simulink model "benchmark_model"  (R2021a)
settings: Solver=ode1  StartTime=0.0  StopTime=Tend  FixedStep=0.0001  MaxStep=0.1  MinStep=0.0001  AbsTol=0.01  EnableMultiTasking=on
undefined symbols (not defined in the file): A1, A2, AL, AM0, AREA, BORE, C_EGR, c_f, c_T, CAIR, cCO, cCO2, cH2, cH2O, cHC, cN2, CO, CO2, cO2, DEN0, DiscIntNeverNeededParam, EGR_dia, EGR_sk, EX_AREA, EX_M_AR, EXO, FD0, FOM, FR0, FR_C1, FR_C2, FR_C3, FR_C4, FR_C5, H2, H2O, HC, INC, INO, KET, Kex, Kh, MAS0, MCh, MHC, MN2, MO2, MOLcylT, N2, O2, PR0, R150, Rabs, SPEC, TBORE, Th_HC, Th_knock, THEX, THIN, TM0 ... (+9)
libraries: pid_lib x1
(part 4 of 6)

== system benchmark_model/ENGINE/engine_s/cylinders/cyl1/cyl/heat_trans/cyl_wall ==
  qw_v : Inport
  Tw0 : Inport  Port=2
  Gain1 : Gain  Gain=1/2.5
  Gain2 : Gain  Gain=1.0
  Gain5 : Gain  Gain=3.0
  Integrator : Integrator  InitialConditionSource=external
  Subtract : Sum  Inputs=-+
  Subtract2 : Sum  Inputs=+-
  Tw : Outport
  wires:
  Tw0/1 -> Subtract2/2, Integrator/2
  Subtract/1 -> Gain1/1
  Gain1/1 -> Integrator/1
  Integrator/1 -> Tw/1, Subtract2/1
  Gain2/1 -> Subtract/2
  Subtract2/1 -> Gain5/1
  Gain5/1 -> Subtract/1
  qw_v/1 -> Gain2/1

== system benchmark_model/ENGINE/engine_s/cylinders/cyl1/cyl/knock_Integral/Subsystem1 ==
  pc : Inport
  rps : Inport  Port=2
  Tc : Inport  Port=3
  rad : Inport  Port=4
  Constant1 : Constant  Value=0
  Constant2 : Constant  Value=FR_C1
  Constant3 : Constant
  Constant4 : Constant  Value=(540+INC)*pi/180
  Constant5 : Constant  Value=(180-EXO)*pi/180
  Divide1 : Product  Inputs=3
  Divide2 : Product  Inputs=*/
  Fcn : Fcn  Expr=-FR_C2*(-FR_C4*u+FR_C5)
  Gain : Gain  Gain=0.001
  Integrator : Integrator  ExternalReset=rising
  Math Function : Math  Operator=pow  SignedPower=on  SaturateOnIntegerOverflow=on
  Memory : Memory
  Relational Operator1 : RelationalOperator  Operator=<=  OutDataTypeStr=boolean  RndMeth=Nearest
  Relational Operator2 : RelationalOperator  OutDataTypeStr=boolean  RndMeth=Nearest
  Saturation : Saturate  UpperLimit=inf  LowerLimit=1.0e-16
  Subsystem : Subsystem
  Switch : Switch  Threshold=0.5
  cal_unburned_temp : Subsystem
  ki : Outport
  wires:
  pc/1 -> Saturation/1
  Fcn/1 -> Math Function/2
  Math Function/1 -> Divide1/2
  Constant2/1 -> Divide1/1
  Subsystem/1(Out1) -> Divide1/3
  Divide1/1 -> Divide2/2
  Constant3/1 -> Divide2/1
  Divide2/1 -> Integrator/1
  Tc/1 -> cal_unburned_temp/2(Tc)
  Memory/1 -> Integrator/2
  cal_unburned_temp/1(Tu) -> Subsystem/1(Tu)
  Gain/1 -> Math Function/1
  Integrator/1 -> Switch/1
  Switch/1 -> ki/1
  Constant1/1 -> Switch/3
  rad/1 -> Relational Operator1/1, Relational Operator2/1
  Constant4/1 -> Relational Operator2/2
  Relational Operator2/1 -> cal_unburned_temp/3(trg_inc), Memory/1
  Constant5/1 -> Relational Operator1/2
  Relational Operator1/1 -> Switch/2
  rps/1 -> Fcn/1
  Saturation/1 -> cal_unburned_temp/1(Pc), Gain/1

== system benchmark_model/ENGINE/engine_s/cylinders/cyl1/cyl/knock_Integral/Triggered Subsystem ==
  QA_max : Inport
  QA : Inport  Port=2
  Trigger : TriggerPort  VariantControl=(inherit)
  Constant1 : Constant  Value=0
  Constant2 : Constant  Value=1.0e-9
  Relational Operator : RelationalOperator  OutDataTypeStr=boolean  RndMeth=Nearest
  Subtract : Sum  Inputs=+-
  Switch : Switch  Threshold=0.5
  AI_Q : Outport  InitialOutput=0
  wires:
  QA/1 -> Subtract/2
  QA_max/1 -> Subtract/1
  Constant1/1 -> Switch/3
  Switch/1 -> AI_Q/1
  Subtract/1 -> Relational Operator/1, Switch/1
  Relational Operator/1 -> Switch/2
  Constant2/1 -> Relational Operator/2

== system benchmark_model/ENGINE/engine_s/cylinders/cyl1/cyl/ramining ratio of fuel/Triggered Subsystem ==
  QA : Inport
  Trigger : TriggerPort  VariantControl=(inherit)
  Constant : Constant
  Constant1 : Constant  Value=0
  Constant2 : Constant  Value=1.0e-9
  Relational Operator : RelationalOperator  OutDataTypeStr=boolean  RndMeth=Nearest
  Subtract : Sum  Inputs=+-
  Switch : Switch  Threshold=0.5
  AI_Q : Outport  InitialOutput=0
  wires:
  Constant2/1 -> Relational Operator/2
  Relational Operator/1 -> Switch/2
  Subtract/1 -> Switch/1, Relational Operator/1
  Switch/1 -> AI_Q/1
  Constant1/1 -> Switch/3
  Constant/1 -> Subtract/1
  QA/1 -> Subtract/2

== system benchmark_model/ENGINE/engine_s/cylinders/cyl1/cyl/unburnt_gass/add_fuel1 ==
  Nfuel : Inport
  mol : Inport  Port=2
  Add : Sum
  Demux : Demux  Outputs=7
  Mux : Mux  Inputs=7
  add_fuel : Outport
  wires:
  Demux/2 -> Mux/2
  Demux/3 -> Mux/3
  Demux/4 -> Mux/4
  Demux/5 -> Mux/5
  Demux/6 -> Mux/6
  Demux/7 -> Mux/7
  mol/1 -> Demux/1
  Mux/1 -> add_fuel/1
  Demux/1 -> Add/2
  Add/1 -> Mux/1
  Nfuel/1 -> Add/1

== system benchmark_model/ENGINE/engine_s/cylinders/cyl1/cyl/unburnt_gass/init&trig ==
  trig : Inport
  value : Inport  Port=2
  Demux : Demux  Outputs=7
  Mux : Mux  Inputs=7
  qChart : Stateflow chart  TreatAsAtomicUnit=on
  init : Outport
  wires:
  value/1 -> Demux/1
  Demux/1 -> qChart/1(sl_in1)
  Demux/2 -> qChart/2(sl_in2)
  Demux/3 -> qChart/3(sl_in3)
  Demux/4 -> qChart/4(sl_in4)
  Demux/5 -> qChart/5(sl_in5)
  Demux/6 -> qChart/6(sl_in6)
  Demux/7 -> qChart/7(sl_in7)
  qChart/7(sl_out7) -> Mux/7
  qChart/1(sl_out1) -> Mux/1
  qChart/2(sl_out2) -> Mux/2
  qChart/3(sl_out3) -> Mux/3
  qChart/4(sl_out4) -> Mux/4
  qChart/5(sl_out5) -> Mux/5
  qChart/6(sl_out6) -> Mux/6
  Mux/1 -> init/1
  trig/1 -> qChart/Trigger

== system benchmark_model/ENGINE/engine_s/cylinders/cyl1/selectors/selector/mod720(u,4*pi) ==
  u : Inport
  Constant7 : Constant  Value=4*pi
  Math Function : Math  Operator=mod  SignedPower=on  SaturateOnIntegerOverflow=on
  y : Outport
  wires:
  Math Function/1 -> y/1
  u/1 -> Math Function/1
  Constant7/1 -> Math Function/2

== system benchmark_model/ENGINE/engine_s/cylinders/cyl2/cyl/Energy_Int/dvol ==
  rad : Inport
  rps : Inport  Port=2
  Product : Product  RndMeth=Zero
  func_d_cylvol(u,SPEC) : Subsystem
  dvol : Outport
  wires:
  func_d_cylvol(u,SPEC)/1(Out1) -> Product/1
  rad/1 -> func_d_cylvol(u,SPEC)/1(In1)
  Product/1 -> dvol/1
  rps/1 -> Product/2

== system benchmark_model/ENGINE/engine_s/cylinders/cyl2/cyl/cal_cyl_state/cal_state ==
  note: p/d = R T
      | T = P/d/R
  m : Inport
  n : Inport  Port=2
  f : Inport  Port=3
  E : Inport  Port=4
  vol : Inport  Port=5
  Fcn : Fcn  Expr=2/u[1]*u[3]/u[2]
  Fcn1 : Fcn  Expr=u[3]/u[1]/(Rabs/u[2])
  Mux : Mux  Inputs=3
  Mux1 : Mux
  Mux2 : Mux  Inputs=3
  Product1 : Product  Inputs=/*  RndMeth=Zero
  Product2 : Product  Inputs=*/  RndMeth=Zero
  Product3 : Product  Inputs=*/  RndMeth=Zero
  pc : Outport  InitialOutput=0
  tc : Outport  Port=2  InitialOutput=0
  cyl_st : Outport  Port=3  InitialOutput=0
  wires:
  Fcn1/1 -> tc/1
  E/1 -> Mux/3
  f/1 -> Product1/2
  n/1 -> Product2/2, Product1/1
  m/1 -> Product3/1, Product2/1
  Mux2/1 -> Fcn1/1
  Product3/1 -> Mux1/1, Mux2/1  "dens"
  Product2/1 -> Mux1/3, Mux2/2  "gas_c"
  Product1/1 -> Mux1/4, Mux/1  "deg of freedom"
  vol/1 -> Product3/2, Mux/2
  Mux1/1 -> cyl_st/1
  Mux/1 -> Fcn/1
  Fcn/1 -> pc/1, Mux2/3, Mux1/2  "pres"

== system benchmark_model/ENGINE/engine_s/cylinders/cyl2/cyl/crank/Subsystem1 ==
  trig_inj : Inport
  fc : Inport  Port=2
  N/s : Inport  Port=3
  Gain : Gain  Gain=MHC
  Integrator : Integrator  ExternalReset=rising
  Product : Product
  Relational Operator1 : RelationalOperator  OutDataTypeStr=boolean  RndMeth=Nearest
  N_fuel : Outport
  wires:
  Gain/1 -> Integrator/1
  N/s/1 -> Gain/1, Product/2
  fc/1 -> Relational Operator1/1
  Relational Operator1/1 -> Product/1
  Integrator/1 -> Relational Operator1/2
  Product/1 -> N_fuel/1
  trig_inj/1 -> Integrator/2

== system benchmark_model/ENGINE/engine_s/cylinders/cyl2/cyl/crank/inj_start ==
  rad : Inport
  Constant3 : Constant  Value=(360-INO+1)*pi/180
  Relational Operator2 : RelationalOperator  OutDataTypeStr=boolean  RndMeth=Nearest
  trig_inj : Outport
  wires:
  Relational Operator2/1 -> trig_inj/1
  rad/1 -> Relational Operator2/1
  Constant3/1 -> Relational Operator2/2

== system benchmark_model/ENGINE/engine_s/cylinders/cyl2/cyl/crank/mol_flow_rate ==
  rps : Inport
  Constant1 : Constant  Value=0.50*pi
  Constant2 : Constant  Value=MHC
  Divide2 : Product  Inputs=*/
  Divide3 : Product  Inputs=*/
  Divide4 : Product  Inputs=*/
  inje/s : Constant  Value=(DEN0*VH/14.5)
  N/s : Outport
  wires:
  Divide2/1 -> Divide3/1
  Divide4/1 -> Divide2/2
  rps/1 -> Divide4/2
  Constant1/1 -> Divide4/1
  inje/s/1 -> Divide2/1
  Divide3/1 -> N/s/1
  Constant2/1 -> Divide3/2

== system benchmark_model/ENGINE/engine_s/cylinders/cyl2/cyl/frame/Init_cyl_gas ==
  tr_inc : Inport
  mol_s : Inport  Port=2
  capture_cyl_state : Subsystem  TreatAsAtomicUnit=on
  init_gas : Outport
  Qmax : Outport  Port=2
  b_comp : Outport  Port=3
  af : Outport  Port=4
  wires:
  tr_inc/1 -> capture_cyl_state/Trigger
  capture_cyl_state/4(af) -> af/1
  capture_cyl_state/1(Qmax) -> Qmax/1
  mol_s/1 -> capture_cyl_state/1(cyl_gas)
  capture_cyl_state/2(b_comp) -> b_comp/1
  capture_cyl_state/3(init_gas) -> init_gas/1

== system benchmark_model/ENGINE/engine_s/cylinders/cyl2/cyl/frame/ratio_burnt1 ==
  rps : Inport
  rad : Inport  Port=2
  AF : Inport  Port=3
  KL : Inport  Port=4
  SA : Inport  Port=5
  EGR : Inport  Port=6
  VT : Inport  Port=7
  Add : Sum
  Constant : Constant  Value=(180-EXO-1)*pi/180+pi
  Constant1 : Constant  Value=0
  Constant2 : Constant  Value=pi
  Constant3 : Constant  Value=0
  Product : Product  RndMeth=Zero
  Relational Operator : RelationalOperator  Operator=<  OutDataTypeStr=boolean  RndMeth=Nearest
  Switch : Switch  Threshold=0.5
  Switch1 : Switch  Threshold=0.5
  mod720(u,4*pi) : Subsystem
  murnt_ratio : Subsystem
  burnt_ratio : Outport  PortDimensions=1  InitialOutput=0
  QR : Outport  Port=2  PortDimensions=1  InitialOutput=0
  Q : Outport  Port=3  PortDimensions=1  InitialOutput=0
  wires:
  VT/1 -> murnt_ratio/7(VT)
  Switch1/1 -> Q/1
  Constant3/1 -> Switch1/3
  murnt_ratio/2(Q) -> Switch1/1
  Constant2/1 -> Add/1
  rad/1 -> Add/2
  Add/1 -> mod720(u,4*pi)/1(u)
  EGR/1 -> murnt_ratio/6(EGR)
  Product/1 -> burnt_ratio/1
  Switch/1 -> QR/1, Product/1
  Constant1/1 -> Switch/3
  Relational Operator/1 -> Switch/2, Switch1/2
  Constant/1 -> Relational Operator/2
  SA/1 -> murnt_ratio/2(SA)
  KL/1 -> murnt_ratio/4(KL)
  AF/1 -> murnt_ratio/5(AF)
  rps/1 -> Product/2, murnt_ratio/3(rps)
  mod720(u,4*pi)/1(y) -> Relational Operator/1, murnt_ratio/1(u)
  murnt_ratio/1(q) -> Switch/1

== system benchmark_model/ENGINE/engine_s/cylinders/cyl2/cyl/heat_trans/cal_cyl_ar ==
  vol : Inport
  Add2 : Sum
  Constant1 : Constant  Value=2*pi*BORE
  Constant2 : Constant  Value=AREA
  Gain1 : Gain  Gain=2
  Product1 : Product  Inputs=*/  RndMeth=Zero
  Product2 : Product  RndMeth=Zero
  cyl_ar : Outport
  wires:
  Product2/1 -> Add2/1
  Constant1/1 -> Product2/1
  Product1/1 -> Product2/2
  Add2/1 -> cyl_ar/1
  vol/1 -> Product1/1
  Gain1/1 -> Add2/2
  Constant2/1 -> Gain1/1, Product1/2

== system benchmark_model/ENGINE/engine_s/cylinders/cyl2/cyl/heat_trans/cal_qw ==
  pc : Inport
  rps : Inport  Port=2
  Tg : Inport  Port=3
  Tw : Inport  Port=4
  Fcn : Fcn  Expr=(u(1)*u(2))^0.786*u(3)^(-0.525)*(u(3)-u(4))
  Mux3 : Mux
  Saturation : Saturate  UpperLimit=inf  LowerLimit=1.0e-16
  qw : Outport
  wires:
  Saturation/1 -> Fcn/1
  Tg/1 -> Mux3/3
  rps/1 -> Mux3/2
  pc/1 -> Mux3/1
  Tw/1 -> Mux3/4
  Fcn/1 -> qw/1
  Mux3/1 -> Saturation/1

== system benchmark_model/ENGINE/engine_s/cylinders/cyl2/cyl/heat_trans/cyl_wall ==
  qw_v : Inport
  Tw0 : Inport  Port=2
  Gain1 : Gain  Gain=1/2.5
  Gain2 : Gain  Gain=1.0
  Gain5 : Gain  Gain=3.0
  Integrator : Integrator  InitialConditionSource=external
  Subtract : Sum  Inputs=-+
  Subtract2 : Sum  Inputs=+-
  Tw : Outport
  wires:
  qw_v/1 -> Gain2/1
  Gain5/1 -> Subtract/1
  Subtract2/1 -> Gain5/1
  Gain2/1 -> Subtract/2
  Integrator/1 -> Subtract2/1, Tw/1
  Gain1/1 -> Integrator/1
  Subtract/1 -> Gain1/1
  Tw0/1 -> Integrator/2, Subtract2/2

== system benchmark_model/ENGINE/engine_s/cylinders/cyl2/cyl/knock_Integral/Subsystem1 ==
  pc : Inport
  rps : Inport  Port=2
  Tc : Inport  Port=3
  rad : Inport  Port=4
  Constant1 : Constant  Value=0
  Constant2 : Constant  Value=FR_C1
  Constant3 : Constant
  Constant4 : Constant  Value=(540+INC)*pi/180
  Constant5 : Constant  Value=(180-EXO)*pi/180
  Divide1 : Product  Inputs=3
  Divide2 : Product  Inputs=*/
  Fcn : Fcn  Expr=-FR_C2*(-FR_C4*u+FR_C5)
  Gain : Gain  Gain=0.001
  Integrator : Integrator  ExternalReset=rising
  Math Function : Math  Operator=pow  SignedPower=on  SaturateOnIntegerOverflow=on
  Memory : Memory
  Relational Operator1 : RelationalOperator  Operator=<=  OutDataTypeStr=boolean  RndMeth=Nearest
  Relational Operator2 : RelationalOperator  OutDataTypeStr=boolean  RndMeth=Nearest
  Saturation : Saturate  UpperLimit=inf  LowerLimit=1.0e-16
  Subsystem : Subsystem
  Switch : Switch  Threshold=0.5
  cal_unburned_temp : Subsystem
  ki : Outport
  wires:
  Saturation/1 -> Gain/1, cal_unburned_temp/1(Pc)
  rps/1 -> Fcn/1
  Relational Operator1/1 -> Switch/2
  Constant5/1 -> Relational Operator1/2
  Relational Operator2/1 -> Memory/1, cal_unburned_temp/3(trg_inc)
  Constant4/1 -> Relational Operator2/2
  rad/1 -> Relational Operator2/1, Relational Operator1/1
  Constant1/1 -> Switch/3
  Switch/1 -> ki/1
  Integrator/1 -> Switch/1
  Gain/1 -> Math Function/1
  cal_unburned_temp/1(Tu) -> Subsystem/1(Tu)
  Memory/1 -> Integrator/2
  Tc/1 -> cal_unburned_temp/2(Tc)
  Divide2/1 -> Integrator/1
  Constant3/1 -> Divide2/1
  Divide1/1 -> Divide2/2
  Subsystem/1(Out1) -> Divide1/3
  Constant2/1 -> Divide1/1
  Math Function/1 -> Divide1/2
  Fcn/1 -> Math Function/2
  pc/1 -> Saturation/1

== system benchmark_model/ENGINE/engine_s/cylinders/cyl2/cyl/knock_Integral/Triggered Subsystem ==
  QA_max : Inport
  QA : Inport  Port=2
  Trigger : TriggerPort  VariantControl=(inherit)
  Constant1 : Constant  Value=0
  Constant2 : Constant  Value=1.0e-9
  Relational Operator : RelationalOperator  OutDataTypeStr=boolean  RndMeth=Nearest
  Subtract : Sum  Inputs=+-
  Switch : Switch  Threshold=0.5
  AI_Q : Outport  InitialOutput=0
  wires:
  Constant2/1 -> Relational Operator/2
  Relational Operator/1 -> Switch/2
  Subtract/1 -> Switch/1, Relational Operator/1
  Switch/1 -> AI_Q/1
  Constant1/1 -> Switch/3
  QA_max/1 -> Subtract/1
  QA/1 -> Subtract/2

== system benchmark_model/ENGINE/engine_s/cylinders/cyl2/cyl/ramining ratio of fuel/Triggered Subsystem ==
  QA : Inport
  Trigger : TriggerPort  VariantControl=(inherit)
  Constant : Constant
  Constant1 : Constant  Value=0
  Constant2 : Constant  Value=1.0e-9
  Relational Operator : RelationalOperator  OutDataTypeStr=boolean  RndMeth=Nearest
  Subtract : Sum  Inputs=+-
  Switch : Switch  Threshold=0.5
  AI_Q : Outport  InitialOutput=0
  wires:
  QA/1 -> Subtract/2
  Constant/1 -> Subtract/1
  Constant1/1 -> Switch/3
  Switch/1 -> AI_Q/1
  Subtract/1 -> Relational Operator/1, Switch/1
  Relational Operator/1 -> Switch/2
  Constant2/1 -> Relational Operator/2

== system benchmark_model/ENGINE/engine_s/cylinders/cyl2/cyl/unburnt_gass/add_fuel1 ==
  Nfuel : Inport
  mol : Inport  Port=2
  Add : Sum
  Demux : Demux  Outputs=7
  Mux : Mux  Inputs=7
  add_fuel : Outport
  wires:
  Nfuel/1 -> Add/1
  Add/1 -> Mux/1
  Demux/1 -> Add/2
  Mux/1 -> add_fuel/1
  mol/1 -> Demux/1
  Demux/7 -> Mux/7
  Demux/6 -> Mux/6
  Demux/5 -> Mux/5
  Demux/4 -> Mux/4
  Demux/3 -> Mux/3
  Demux/2 -> Mux/2

== system benchmark_model/ENGINE/engine_s/cylinders/cyl2/cyl/unburnt_gass/init&trig ==
  trig : Inport
  value : Inport  Port=2
  Demux : Demux  Outputs=7
  Mux : Mux  Inputs=7
  qChart : Stateflow chart  TreatAsAtomicUnit=on
  init : Outport
  wires:
  trig/1 -> qChart/Trigger
  Mux/1 -> init/1
  qChart/6(sl_out6) -> Mux/6
  qChart/5(sl_out5) -> Mux/5
  qChart/4(sl_out4) -> Mux/4
  qChart/3(sl_out3) -> Mux/3
  qChart/2(sl_out2) -> Mux/2
  qChart/1(sl_out1) -> Mux/1
  qChart/7(sl_out7) -> Mux/7
  Demux/7 -> qChart/7(sl_in7)
  Demux/6 -> qChart/6(sl_in6)
  Demux/5 -> qChart/5(sl_in5)
  Demux/4 -> qChart/4(sl_in4)
  Demux/3 -> qChart/3(sl_in3)
  Demux/2 -> qChart/2(sl_in2)
  Demux/1 -> qChart/1(sl_in1)
  value/1 -> Demux/1

== system benchmark_model/ENGINE/engine_s/cylinders/cyl2/selectors/selector/mod720(u,4*pi) ==
  u : Inport
  Constant7 : Constant  Value=4*pi
  Math Function : Math  Operator=mod  SignedPower=on  SaturateOnIntegerOverflow=on
  y : Outport
  wires:
  Constant7/1 -> Math Function/2
  u/1 -> Math Function/1
  Math Function/1 -> y/1

== system benchmark_model/ENGINE/engine_s/cylinders/cyl3/cyl/Energy_Int/dvol ==
  rad : Inport
  rps : Inport  Port=2
  Product : Product  RndMeth=Zero
  func_d_cylvol(u,SPEC) : Subsystem
  dvol : Outport
  wires:
  rps/1 -> Product/2
  Product/1 -> dvol/1
  rad/1 -> func_d_cylvol(u,SPEC)/1(In1)
  func_d_cylvol(u,SPEC)/1(Out1) -> Product/1

== system benchmark_model/ENGINE/engine_s/cylinders/cyl3/cyl/cal_cyl_state/cal_state ==
  note: p/d = R T
      | T = P/d/R
  m : Inport
  n : Inport  Port=2
  f : Inport  Port=3
  E : Inport  Port=4
  vol : Inport  Port=5
  Fcn : Fcn  Expr=2/u[1]*u[3]/u[2]
  Fcn1 : Fcn  Expr=u[3]/u[1]/(Rabs/u[2])
  Mux : Mux  Inputs=3
  Mux1 : Mux
  Mux2 : Mux  Inputs=3
  Product1 : Product  Inputs=/*  RndMeth=Zero
  Product2 : Product  Inputs=*/  RndMeth=Zero
  Product3 : Product  Inputs=*/  RndMeth=Zero
  pc : Outport  InitialOutput=0
  tc : Outport  Port=2  InitialOutput=0
  cyl_st : Outport  Port=3  InitialOutput=0
  wires:
  Fcn/1 -> Mux1/2, Mux2/3, pc/1  "pres"
  Mux/1 -> Fcn/1
  Mux1/1 -> cyl_st/1
  vol/1 -> Mux/2, Product3/2
  Product1/1 -> Mux/1, Mux1/4  "deg of freedom"
  Product2/1 -> Mux2/2, Mux1/3  "gas_c"
  Product3/1 -> Mux2/1, Mux1/1  "dens"
  Mux2/1 -> Fcn1/1
  m/1 -> Product2/1, Product3/1
  n/1 -> Product1/1, Product2/2
  f/1 -> Product1/2
  E/1 -> Mux/3
  Fcn1/1 -> tc/1

== system benchmark_model/ENGINE/engine_s/cylinders/cyl3/cyl/crank/Subsystem1 ==
  trig_inj : Inport
  fc : Inport  Port=2
  N/s : Inport  Port=3
  Gain : Gain  Gain=MHC
  Integrator : Integrator  ExternalReset=rising
  Product : Product
  Relational Operator1 : RelationalOperator  OutDataTypeStr=boolean  RndMeth=Nearest
  N_fuel : Outport
  wires:
  trig_inj/1 -> Integrator/2
  Product/1 -> N_fuel/1
  Integrator/1 -> Relational Operator1/2
  Relational Operator1/1 -> Product/1
  fc/1 -> Relational Operator1/1
  N/s/1 -> Product/2, Gain/1
  Gain/1 -> Integrator/1

== system benchmark_model/ENGINE/engine_s/cylinders/cyl3/cyl/crank/inj_start ==
  rad : Inport
  Constant3 : Constant  Value=(360-INO+1)*pi/180
  Relational Operator2 : RelationalOperator  OutDataTypeStr=boolean  RndMeth=Nearest
  trig_inj : Outport
  wires:
  Constant3/1 -> Relational Operator2/2
  rad/1 -> Relational Operator2/1
  Relational Operator2/1 -> trig_inj/1

== system benchmark_model/ENGINE/engine_s/cylinders/cyl3/cyl/crank/mol_flow_rate ==
  rps : Inport
  Constant1 : Constant  Value=0.50*pi
  Constant2 : Constant  Value=MHC
  Divide2 : Product  Inputs=*/
  Divide3 : Product  Inputs=*/
  Divide4 : Product  Inputs=*/
  inje/s : Constant  Value=(DEN0*VH/14.5)
  N/s : Outport
  wires:
  Constant2/1 -> Divide3/2
  Divide3/1 -> N/s/1
  inje/s/1 -> Divide2/1
  Constant1/1 -> Divide4/1
  rps/1 -> Divide4/2
  Divide4/1 -> Divide2/2
  Divide2/1 -> Divide3/1

== system benchmark_model/ENGINE/engine_s/cylinders/cyl3/cyl/frame/Init_cyl_gas ==
  tr_inc : Inport
  mol_s : Inport  Port=2
  capture_cyl_state : Subsystem  TreatAsAtomicUnit=on
  init_gas : Outport
  Qmax : Outport  Port=2
  b_comp : Outport  Port=3
  af : Outport  Port=4
  wires:
  capture_cyl_state/3(init_gas) -> init_gas/1
  capture_cyl_state/2(b_comp) -> b_comp/1
  mol_s/1 -> capture_cyl_state/1(cyl_gas)
  capture_cyl_state/1(Qmax) -> Qmax/1
  capture_cyl_state/4(af) -> af/1
  tr_inc/1 -> capture_cyl_state/Trigger

== system benchmark_model/ENGINE/engine_s/cylinders/cyl3/cyl/frame/ratio_burnt1 ==
  rps : Inport
  rad : Inport  Port=2
  AF : Inport  Port=3
  KL : Inport  Port=4
  SA : Inport  Port=5
  EGR : Inport  Port=6
  VT : Inport  Port=7
  Add : Sum
  Constant : Constant  Value=(180-EXO-1)*pi/180+pi
  Constant1 : Constant  Value=0
  Constant2 : Constant  Value=pi
  Constant3 : Constant  Value=0
  Product : Product  RndMeth=Zero
  Relational Operator : RelationalOperator  Operator=<  OutDataTypeStr=boolean  RndMeth=Nearest
  Switch : Switch  Threshold=0.5
  Switch1 : Switch  Threshold=0.5
  mod720(u,4*pi) : Subsystem
  murnt_ratio : Subsystem
  burnt_ratio : Outport  PortDimensions=1  InitialOutput=0
  QR : Outport  Port=2  PortDimensions=1  InitialOutput=0
  Q : Outport  Port=3  PortDimensions=1  InitialOutput=0
  wires:
  murnt_ratio/1(q) -> Switch/1
  mod720(u,4*pi)/1(y) -> murnt_ratio/1(u), Relational Operator/1
  rps/1 -> murnt_ratio/3(rps), Product/2
  AF/1 -> murnt_ratio/5(AF)
  KL/1 -> murnt_ratio/4(KL)
  SA/1 -> murnt_ratio/2(SA)
  Constant/1 -> Relational Operator/2
  Relational Operator/1 -> Switch1/2, Switch/2
  Constant1/1 -> Switch/3
  Switch/1 -> Product/1, QR/1
  Product/1 -> burnt_ratio/1
  EGR/1 -> murnt_ratio/6(EGR)
  Add/1 -> mod720(u,4*pi)/1(u)
  rad/1 -> Add/2
  Constant2/1 -> Add/1
  murnt_ratio/2(Q) -> Switch1/1
  Constant3/1 -> Switch1/3
  Switch1/1 -> Q/1
  VT/1 -> murnt_ratio/7(VT)

== system benchmark_model/ENGINE/engine_s/cylinders/cyl3/cyl/heat_trans/cal_cyl_ar ==
  vol : Inport
  Add2 : Sum
  Constant1 : Constant  Value=2*pi*BORE
  Constant2 : Constant  Value=AREA
  Gain1 : Gain  Gain=2
  Product1 : Product  Inputs=*/  RndMeth=Zero
  Product2 : Product  RndMeth=Zero
  cyl_ar : Outport
  wires:
  Constant2/1 -> Product1/2, Gain1/1
  Gain1/1 -> Add2/2
  vol/1 -> Product1/1
  Add2/1 -> cyl_ar/1
  Product1/1 -> Product2/2
  Constant1/1 -> Product2/1
  Product2/1 -> Add2/1

== system benchmark_model/ENGINE/engine_s/cylinders/cyl3/cyl/heat_trans/cal_qw ==
  pc : Inport
  rps : Inport  Port=2
  Tg : Inport  Port=3
  Tw : Inport  Port=4
  Fcn : Fcn  Expr=(u(1)*u(2))^0.786*u(3)^(-0.525)*(u(3)-u(4))
  Mux3 : Mux
  Saturation : Saturate  UpperLimit=inf  LowerLimit=1.0e-16
  qw : Outport
  wires:
  Mux3/1 -> Saturation/1
  Fcn/1 -> qw/1
  Tw/1 -> Mux3/4
  pc/1 -> Mux3/1
  rps/1 -> Mux3/2
  Tg/1 -> Mux3/3
  Saturation/1 -> Fcn/1

== system benchmark_model/ENGINE/engine_s/cylinders/cyl3/cyl/heat_trans/cyl_wall ==
  qw_v : Inport
  Tw0 : Inport  Port=2
  Gain1 : Gain  Gain=1/2.5
  Gain2 : Gain  Gain=1.0
  Gain5 : Gain  Gain=3.0
  Integrator : Integrator  InitialConditionSource=external
  Subtract : Sum  Inputs=-+
  Subtract2 : Sum  Inputs=+-
  Tw : Outport
  wires:
  Tw0/1 -> Subtract2/2, Integrator/2
  Subtract/1 -> Gain1/1
  Gain1/1 -> Integrator/1
  Integrator/1 -> Tw/1, Subtract2/1
  Gain2/1 -> Subtract/2
  Subtract2/1 -> Gain5/1
  Gain5/1 -> Subtract/1
  qw_v/1 -> Gain2/1

== system benchmark_model/ENGINE/engine_s/cylinders/cyl3/cyl/knock_Integral/Subsystem1 ==
  pc : Inport
  rps : Inport  Port=2
  Tc : Inport  Port=3
  rad : Inport  Port=4
  Constant1 : Constant  Value=0
  Constant2 : Constant  Value=FR_C1
  Constant3 : Constant
  Constant4 : Constant  Value=(540+INC)*pi/180
  Constant5 : Constant  Value=(180-EXO)*pi/180
  Divide1 : Product  Inputs=3
  Divide2 : Product  Inputs=*/
  Fcn : Fcn  Expr=-FR_C2*(-FR_C4*u+FR_C5)
  Gain : Gain  Gain=0.001
  Integrator : Integrator  ExternalReset=rising
  Math Function : Math  Operator=pow  SignedPower=on  SaturateOnIntegerOverflow=on
  Memory : Memory
  Relational Operator1 : RelationalOperator  Operator=<=  OutDataTypeStr=boolean  RndMeth=Nearest
  Relational Operator2 : RelationalOperator  OutDataTypeStr=boolean  RndMeth=Nearest
  Saturation : Saturate  UpperLimit=inf  LowerLimit=1.0e-16
  Subsystem : Subsystem
  Switch : Switch  Threshold=0.5
  cal_unburned_temp : Subsystem
  ki : Outport
  wires:
  pc/1 -> Saturation/1
  Fcn/1 -> Math Function/2
  Math Function/1 -> Divide1/2
  Constant2/1 -> Divide1/1
  Subsystem/1(Out1) -> Divide1/3
  Divide1/1 -> Divide2/2
  Constant3/1 -> Divide2/1
  Divide2/1 -> Integrator/1
  Tc/1 -> cal_unburned_temp/2(Tc)
  Memory/1 -> Integrator/2
  cal_unburned_temp/1(Tu) -> Subsystem/1(Tu)
  Gain/1 -> Math Function/1
  Integrator/1 -> Switch/1
  Switch/1 -> ki/1
  Constant1/1 -> Switch/3
  rad/1 -> Relational Operator1/1, Relational Operator2/1
  Constant4/1 -> Relational Operator2/2
  Relational Operator2/1 -> cal_unburned_temp/3(trg_inc), Memory/1
  Constant5/1 -> Relational Operator1/2
  Relational Operator1/1 -> Switch/2
  rps/1 -> Fcn/1
  Saturation/1 -> cal_unburned_temp/1(Pc), Gain/1

== system benchmark_model/ENGINE/engine_s/cylinders/cyl3/cyl/knock_Integral/Triggered Subsystem ==
  QA_max : Inport
  QA : Inport  Port=2
  Trigger : TriggerPort  VariantControl=(inherit)
  Constant1 : Constant  Value=0
  Constant2 : Constant  Value=1.0e-9
  Relational Operator : RelationalOperator  OutDataTypeStr=boolean  RndMeth=Nearest
  Subtract : Sum  Inputs=+-
  Switch : Switch  Threshold=0.5
  AI_Q : Outport  InitialOutput=0
  wires:
  QA/1 -> Subtract/2
  QA_max/1 -> Subtract/1
  Constant1/1 -> Switch/3
  Switch/1 -> AI_Q/1
  Subtract/1 -> Relational Operator/1, Switch/1
  Relational Operator/1 -> Switch/2
  Constant2/1 -> Relational Operator/2

== system benchmark_model/ENGINE/engine_s/cylinders/cyl3/cyl/ramining ratio of fuel/Triggered Subsystem ==
  QA : Inport
  Trigger : TriggerPort  VariantControl=(inherit)
  Constant : Constant
  Constant1 : Constant  Value=0
  Constant2 : Constant  Value=1.0e-9
  Relational Operator : RelationalOperator  OutDataTypeStr=boolean  RndMeth=Nearest
  Subtract : Sum  Inputs=+-
  Switch : Switch  Threshold=0.5
  AI_Q : Outport  InitialOutput=0
  wires:
  Constant2/1 -> Relational Operator/2
  Relational Operator/1 -> Switch/2
  Subtract/1 -> Switch/1, Relational Operator/1
  Switch/1 -> AI_Q/1
  Constant1/1 -> Switch/3
  Constant/1 -> Subtract/1
  QA/1 -> Subtract/2

== system benchmark_model/ENGINE/engine_s/cylinders/cyl3/cyl/unburnt_gass/add_fuel1 ==
  Nfuel : Inport
  mol : Inport  Port=2
  Add : Sum
  Demux : Demux  Outputs=7
  Mux : Mux  Inputs=7
  add_fuel : Outport
  wires:
  Demux/2 -> Mux/2
  Demux/3 -> Mux/3
  Demux/4 -> Mux/4
  Demux/5 -> Mux/5
  Demux/6 -> Mux/6
  Demux/7 -> Mux/7
  mol/1 -> Demux/1
  Mux/1 -> add_fuel/1
  Demux/1 -> Add/2
  Add/1 -> Mux/1
  Nfuel/1 -> Add/1

== system benchmark_model/ENGINE/engine_s/cylinders/cyl3/cyl/unburnt_gass/init&trig ==
  trig : Inport
  value : Inport  Port=2
  Demux : Demux  Outputs=7
  Mux : Mux  Inputs=7
  qChart : Stateflow chart  TreatAsAtomicUnit=on
  init : Outport
  wires:
  value/1 -> Demux/1
  Demux/1 -> qChart/1(sl_in1)
  Demux/2 -> qChart/2(sl_in2)
  Demux/3 -> qChart/3(sl_in3)
  Demux/4 -> qChart/4(sl_in4)
  Demux/5 -> qChart/5(sl_in5)
  Demux/6 -> qChart/6(sl_in6)
  Demux/7 -> qChart/7(sl_in7)
  qChart/7(sl_out7) -> Mux/7
  qChart/1(sl_out1) -> Mux/1
  qChart/2(sl_out2) -> Mux/2
  qChart/3(sl_out3) -> Mux/3
  qChart/4(sl_out4) -> Mux/4
  qChart/5(sl_out5) -> Mux/5
  qChart/6(sl_out6) -> Mux/6
  Mux/1 -> init/1
  trig/1 -> qChart/Trigger

== system benchmark_model/ENGINE/engine_s/cylinders/cyl3/selectors/selector/mod720(u,4*pi) ==
  u : Inport
  Constant7 : Constant  Value=4*pi
  Math Function : Math  Operator=mod  SignedPower=on  SaturateOnIntegerOverflow=on
  y : Outport
  wires:
  Math Function/1 -> y/1
  u/1 -> Math Function/1
  Constant7/1 -> Math Function/2

== system benchmark_model/ENGINE/engine_s/cylinders/cyl4/cyl/Energy_Int/dvol ==
  rad : Inport
  rps : Inport  Port=2
  Product : Product  RndMeth=Zero
  func_d_cylvol(u,SPEC) : Subsystem
  dvol : Outport
  wires:
  func_d_cylvol(u,SPEC)/1(Out1) -> Product/1
  rad/1 -> func_d_cylvol(u,SPEC)/1(In1)
  Product/1 -> dvol/1
  rps/1 -> Product/2

== system benchmark_model/ENGINE/engine_s/cylinders/cyl4/cyl/cal_cyl_state/cal_state ==
  note: p/d = R T
      | T = P/d/R
  m : Inport
  n : Inport  Port=2
  f : Inport  Port=3
  E : Inport  Port=4
  vol : Inport  Port=5
  Fcn : Fcn  Expr=2/u[1]*u[3]/u[2]
  Fcn1 : Fcn  Expr=u[3]/u[1]/(Rabs/u[2])
  Mux : Mux  Inputs=3
  Mux1 : Mux
  Mux2 : Mux  Inputs=3
  Product1 : Product  Inputs=/*  RndMeth=Zero
  Product2 : Product  Inputs=*/  RndMeth=Zero
  Product3 : Product  Inputs=*/  RndMeth=Zero
  pc : Outport  InitialOutput=0
  tc : Outport  Port=2  InitialOutput=0
  cyl_st : Outport  Port=3  InitialOutput=0
  wires:
  Fcn1/1 -> tc/1
  E/1 -> Mux/3
  f/1 -> Product1/2
  n/1 -> Product2/2, Product1/1
  m/1 -> Product3/1, Product2/1
  Mux2/1 -> Fcn1/1
  Product3/1 -> Mux1/1, Mux2/1  "dens"
  Product2/1 -> Mux1/3, Mux2/2  "gas_c"
  Product1/1 -> Mux1/4, Mux/1  "deg of freedom"
  vol/1 -> Product3/2, Mux/2
  Mux1/1 -> cyl_st/1
  Mux/1 -> Fcn/1
  Fcn/1 -> pc/1, Mux2/3, Mux1/2  "pres"

== system benchmark_model/ENGINE/engine_s/cylinders/cyl4/cyl/crank/Subsystem1 ==
  trig_inj : Inport
  fc : Inport  Port=2
  N/s : Inport  Port=3
  Gain : Gain  Gain=MHC
  Integrator : Integrator  ExternalReset=rising
  Product : Product
  Relational Operator1 : RelationalOperator  OutDataTypeStr=boolean  RndMeth=Nearest
  N_fuel : Outport
  wires:
  Gain/1 -> Integrator/1
  N/s/1 -> Gain/1, Product/2
  fc/1 -> Relational Operator1/1
  Relational Operator1/1 -> Product/1
  Integrator/1 -> Relational Operator1/2
  Product/1 -> N_fuel/1
  trig_inj/1 -> Integrator/2

== system benchmark_model/ENGINE/engine_s/cylinders/cyl4/cyl/crank/inj_start ==
  rad : Inport
  Constant3 : Constant  Value=(360-INO+1)*pi/180
  Relational Operator2 : RelationalOperator  OutDataTypeStr=boolean  RndMeth=Nearest
  trig_inj : Outport
  wires:
  Relational Operator2/1 -> trig_inj/1
  rad/1 -> Relational Operator2/1
  Constant3/1 -> Relational Operator2/2

== system benchmark_model/ENGINE/engine_s/cylinders/cyl4/cyl/crank/mol_flow_rate ==
  rps : Inport
  Constant1 : Constant  Value=0.50*pi
  Constant2 : Constant  Value=MHC
  Divide2 : Product  Inputs=*/
  Divide3 : Product  Inputs=*/
  Divide4 : Product  Inputs=*/
  inje/s : Constant  Value=(DEN0*VH/14.5)
  N/s : Outport
  wires:
  Divide2/1 -> Divide3/1
  Divide4/1 -> Divide2/2
  rps/1 -> Divide4/2
  Constant1/1 -> Divide4/1
  inje/s/1 -> Divide2/1
  Divide3/1 -> N/s/1
  Constant2/1 -> Divide3/2

== system benchmark_model/ENGINE/engine_s/cylinders/cyl4/cyl/frame/Init_cyl_gas ==
  tr_inc : Inport
  mol_s : Inport  Port=2
  capture_cyl_state : Subsystem  TreatAsAtomicUnit=on
  init_gas : Outport
  Qmax : Outport  Port=2
  b_comp : Outport  Port=3
  af : Outport  Port=4
  wires:
  tr_inc/1 -> capture_cyl_state/Trigger
  capture_cyl_state/4(af) -> af/1
  capture_cyl_state/1(Qmax) -> Qmax/1
  mol_s/1 -> capture_cyl_state/1(cyl_gas)
  capture_cyl_state/2(b_comp) -> b_comp/1
  capture_cyl_state/3(init_gas) -> init_gas/1

== system benchmark_model/ENGINE/engine_s/cylinders/cyl4/cyl/frame/ratio_burnt1 ==
  rps : Inport
  rad : Inport  Port=2
  AF : Inport  Port=3
  KL : Inport  Port=4
  SA : Inport  Port=5
  EGR : Inport  Port=6
  VT : Inport  Port=7
  Add : Sum
  Constant : Constant  Value=(180-EXO-1)*pi/180+pi
  Constant1 : Constant  Value=0
  Constant2 : Constant  Value=pi
  Constant3 : Constant  Value=0
  Product : Product  RndMeth=Zero
  Relational Operator : RelationalOperator  Operator=<  OutDataTypeStr=boolean  RndMeth=Nearest
  Switch : Switch  Threshold=0.5
  Switch1 : Switch  Threshold=0.5
  mod720(u,4*pi) : Subsystem
  murnt_ratio : Subsystem
  burnt_ratio : Outport  PortDimensions=1  InitialOutput=0
  QR : Outport  Port=2  PortDimensions=1  InitialOutput=0
  Q : Outport  Port=3  PortDimensions=1  InitialOutput=0
  wires:
  VT/1 -> murnt_ratio/7(VT)
  Switch1/1 -> Q/1
  Constant3/1 -> Switch1/3
  murnt_ratio/2(Q) -> Switch1/1
  Constant2/1 -> Add/1
  rad/1 -> Add/2
  Add/1 -> mod720(u,4*pi)/1(u)
  EGR/1 -> murnt_ratio/6(EGR)
  Product/1 -> burnt_ratio/1
  Switch/1 -> QR/1, Product/1
  Constant1/1 -> Switch/3
  Relational Operator/1 -> Switch/2, Switch1/2
  Constant/1 -> Relational Operator/2
  SA/1 -> murnt_ratio/2(SA)
  KL/1 -> murnt_ratio/4(KL)
  AF/1 -> murnt_ratio/5(AF)
  rps/1 -> Product/2, murnt_ratio/3(rps)
  mod720(u,4*pi)/1(y) -> Relational Operator/1, murnt_ratio/1(u)
  murnt_ratio/1(q) -> Switch/1

== system benchmark_model/ENGINE/engine_s/cylinders/cyl4/cyl/heat_trans/cal_cyl_ar ==
  vol : Inport
  Add2 : Sum
  Constant1 : Constant  Value=2*pi*BORE
  Constant2 : Constant  Value=AREA
  Gain1 : Gain  Gain=2
  Product1 : Product  Inputs=*/  RndMeth=Zero
  Product2 : Product  RndMeth=Zero
  cyl_ar : Outport
  wires:
  Product2/1 -> Add2/1
  Constant1/1 -> Product2/1
  Product1/1 -> Product2/2
  Add2/1 -> cyl_ar/1
  vol/1 -> Product1/1
  Gain1/1 -> Add2/2
  Constant2/1 -> Gain1/1, Product1/2

== system benchmark_model/ENGINE/engine_s/cylinders/cyl4/cyl/heat_trans/cal_qw ==
  pc : Inport
  rps : Inport  Port=2
  Tg : Inport  Port=3
  Tw : Inport  Port=4
  Fcn : Fcn  Expr=(u(1)*u(2))^0.786*u(3)^(-0.525)*(u(3)-u(4))
  Mux3 : Mux
  Saturation : Saturate  UpperLimit=inf  LowerLimit=1.0e-16
  qw : Outport
  wires:
  Saturation/1 -> Fcn/1
  Tg/1 -> Mux3/3
  rps/1 -> Mux3/2
  pc/1 -> Mux3/1
  Tw/1 -> Mux3/4
  Fcn/1 -> qw/1
  Mux3/1 -> Saturation/1

== system benchmark_model/ENGINE/engine_s/cylinders/cyl4/cyl/heat_trans/cyl_wall ==
  qw_v : Inport
  Tw0 : Inport  Port=2
  Gain1 : Gain  Gain=1/2.5
  Gain2 : Gain  Gain=1.0
  Gain5 : Gain  Gain=3.0
  Integrator : Integrator  InitialConditionSource=external
  Subtract : Sum  Inputs=-+
  Subtract2 : Sum  Inputs=+-
  Tw : Outport
  wires:
  qw_v/1 -> Gain2/1
  Gain5/1 -> Subtract/1
  Subtract2/1 -> Gain5/1
  Gain2/1 -> Subtract/2
  Integrator/1 -> Subtract2/1, Tw/1
  Gain1/1 -> Integrator/1
  Subtract/1 -> Gain1/1
  Tw0/1 -> Integrator/2, Subtract2/2

== system benchmark_model/ENGINE/engine_s/cylinders/cyl4/cyl/knock_Integral/Subsystem1 ==
  pc : Inport
  rps : Inport  Port=2
  Tc : Inport  Port=3
  rad : Inport  Port=4
  Constant1 : Constant  Value=0
  Constant2 : Constant  Value=FR_C1
  Constant3 : Constant
  Constant4 : Constant  Value=(540+INC)*pi/180
  Constant5 : Constant  Value=(180-EXO)*pi/180
  Divide1 : Product  Inputs=3
  Divide2 : Product  Inputs=*/
  Fcn : Fcn  Expr=-FR_C2*(-FR_C4*u+FR_C5)
  Gain : Gain  Gain=0.001
  Integrator : Integrator  ExternalReset=rising
  Math Function : Math  Operator=pow  SignedPower=on  SaturateOnIntegerOverflow=on
  Memory : Memory
  Relational Operator1 : RelationalOperator  Operator=<=  OutDataTypeStr=boolean  RndMeth=Nearest
  Relational Operator2 : RelationalOperator  OutDataTypeStr=boolean  RndMeth=Nearest
  Saturation : Saturate  UpperLimit=inf  LowerLimit=1.0e-16
  Subsystem : Subsystem
  Switch : Switch  Threshold=0.5
  cal_unburned_temp : Subsystem
  ki : Outport
  wires:
  Saturation/1 -> Gain/1, cal_unburned_temp/1(Pc)
  rps/1 -> Fcn/1
  Relational Operator1/1 -> Switch/2
  Constant5/1 -> Relational Operator1/2
  Relational Operator2/1 -> Memory/1, cal_unburned_temp/3(trg_inc)
  Constant4/1 -> Relational Operator2/2
  rad/1 -> Relational Operator2/1, Relational Operator1/1
  Constant1/1 -> Switch/3
  Switch/1 -> ki/1
  Integrator/1 -> Switch/1
  Gain/1 -> Math Function/1
  cal_unburned_temp/1(Tu) -> Subsystem/1(Tu)
  Memory/1 -> Integrator/2
  Tc/1 -> cal_unburned_temp/2(Tc)
  Divide2/1 -> Integrator/1
  Constant3/1 -> Divide2/1
  Divide1/1 -> Divide2/2
  Subsystem/1(Out1) -> Divide1/3
  Constant2/1 -> Divide1/1
  Math Function/1 -> Divide1/2
  Fcn/1 -> Math Function/2
  pc/1 -> Saturation/1

== system benchmark_model/ENGINE/engine_s/cylinders/cyl4/cyl/knock_Integral/Triggered Subsystem ==
  QA_max : Inport
  QA : Inport  Port=2
  Trigger : TriggerPort  VariantControl=(inherit)
  Constant1 : Constant  Value=0
  Constant2 : Constant  Value=1.0e-9
  Relational Operator : RelationalOperator  OutDataTypeStr=boolean  RndMeth=Nearest
  Subtract : Sum  Inputs=+-
  Switch : Switch  Threshold=0.5
  AI_Q : Outport  InitialOutput=0
  wires:
  Constant2/1 -> Relational Operator/2
  Relational Operator/1 -> Switch/2
  Subtract/1 -> Switch/1, Relational Operator/1
  Switch/1 -> AI_Q/1
  Constant1/1 -> Switch/3
  QA_max/1 -> Subtract/1
  QA/1 -> Subtract/2

== system benchmark_model/ENGINE/engine_s/cylinders/cyl4/cyl/ramining ratio of fuel/Triggered Subsystem ==
  QA : Inport
  Trigger : TriggerPort  VariantControl=(inherit)
  Constant : Constant
  Constant1 : Constant  Value=0
  Constant2 : Constant  Value=1.0e-9
  Relational Operator : RelationalOperator  OutDataTypeStr=boolean  RndMeth=Nearest
  Subtract : Sum  Inputs=+-
  Switch : Switch  Threshold=0.5
  AI_Q : Outport  InitialOutput=0
  wires:
  QA/1 -> Subtract/2
  Constant/1 -> Subtract/1
  Constant1/1 -> Switch/3
  Switch/1 -> AI_Q/1
  Subtract/1 -> Relational Operator/1, Switch/1
  Relational Operator/1 -> Switch/2
  Constant2/1 -> Relational Operator/2

== system benchmark_model/ENGINE/engine_s/cylinders/cyl4/cyl/unburnt_gass/add_fuel1 ==
  Nfuel : Inport
  mol : Inport  Port=2
  Add : Sum
  Demux : Demux  Outputs=7
  Mux : Mux  Inputs=7
  add_fuel : Outport
  wires:
  Nfuel/1 -> Add/1
  Add/1 -> Mux/1
  Demux/1 -> Add/2
  Mux/1 -> add_fuel/1
  mol/1 -> Demux/1
  Demux/7 -> Mux/7
  Demux/6 -> Mux/6
  Demux/5 -> Mux/5
  Demux/4 -> Mux/4
  Demux/3 -> Mux/3
  Demux/2 -> Mux/2

== system benchmark_model/ENGINE/engine_s/cylinders/cyl4/cyl/unburnt_gass/init&trig ==
  trig : Inport
  value : Inport  Port=2
  Demux : Demux  Outputs=7
  Mux : Mux  Inputs=7
  qChart : Stateflow chart  TreatAsAtomicUnit=on
  init : Outport
  wires:
  trig/1 -> qChart/Trigger
  Mux/1 -> init/1
  qChart/6(sl_out6) -> Mux/6
  qChart/5(sl_out5) -> Mux/5
  qChart/4(sl_out4) -> Mux/4
  qChart/3(sl_out3) -> Mux/3
  qChart/2(sl_out2) -> Mux/2
  qChart/1(sl_out1) -> Mux/1
  qChart/7(sl_out7) -> Mux/7
  Demux/7 -> qChart/7(sl_in7)
  Demux/6 -> qChart/6(sl_in6)
  Demux/5 -> qChart/5(sl_in5)
  Demux/4 -> qChart/4(sl_in4)
  Demux/3 -> qChart/3(sl_in3)
  Demux/2 -> qChart/2(sl_in2)
  Demux/1 -> qChart/1(sl_in1)
  value/1 -> Demux/1

== system benchmark_model/ENGINE/engine_s/cylinders/cyl4/selectors/selector/mod720(u,4*pi) ==
  u : Inport
  Constant7 : Constant  Value=4*pi
  Math Function : Math  Operator=mod  SignedPower=on  SaturateOnIntegerOverflow=on
  y : Outport
  wires:
  Constant7/1 -> Math Function/2
  u/1 -> Math Function/1
  Math Function/1 -> y/1

== system benchmark_model/ENGINE/engine_s/cylinders/cyl1/cyl/Energy_Int/dvol/func_d_cylvol(u,SPEC) ==
  In1 : Inport
  Constant1 : Constant  Value=SPEC
  Embedded MATLAB Function1 : MATLAB Function  TreatAsAtomicUnit=on
  Out1 : Outport
  wires:
  Constant1/1 -> Embedded MATLAB Function1/2(SPEC)
  In1/1 -> Embedded MATLAB Function1/1(u)
  Embedded MATLAB Function1/1(y) -> Out1/1

== system benchmark_model/ENGINE/engine_s/cylinders/cyl1/cyl/frame/Init_cyl_gas/capture_cyl_state ==
  cyl_gas : Inport
  Trigger : TriggerPort  VariantControl=(inherit)
  Add : Sum  Inputs=++++
  C+O2->CO2 : Constant  Value=4.19*97200.0
  CO+1/2O2->CO2 : Constant  Value=4.19*29620.0
  H+1/2O2->H2O : Constant  Value=4.19*57750.0
  H+1/2O2->H2O1 : Constant  Value=4.19*57750.0
  H/C : Constant  Value=y/2
  Product : Product  RndMeth=Zero
  Product1 : Product  RndMeth=Zero
  Product2 : Product  RndMeth=Zero
  Product3 : Product  Inputs=3  RndMeth=Zero
  Saturation : Saturate  UpperLimit=22  LowerLimit=6
  Selector1 : Selector  InputPortWidth=7  IndexOptions=Index vector (dialog)  Indices=[3]  OutputSizes=[(-2)]
  Selector2 : Selector  InputPortWidth=7  IndexOptions=Index vector (dialog)  Indices=[5]  OutputSizes=[(-2)]
  Selector3 : Selector  InputPortWidth=7  IndexOptions=Index vector (dialog)  Indices=[1]  OutputSizes=[(-2)]
  Selector4 : Selector  InputPortWidth=7  IndexOptions=Index vector (dialog)  Indices=[1]  OutputSizes=[(-2)]
  Subtract : Sum  Inputs=-+
  burnt_compsition : Subsystem
  cal_af : Subsystem
  Qmax : Outport
  b_comp : Outport  Port=2  InitialOutput=[0;0;0;0;0;0;0]
  init_gas : Outport  Port=3  InitialOutput=[0;0;0;0;0;0;0]
  af : Outport  Port=4  InitialOutput=0
  wires:
  Subtract/1 -> Selector3/1, Selector2/1, Selector1/1, Selector4/1
  Add/1 -> Qmax/1
  H+1/2O2->H2O/1 -> Product2/2
  Selector2/1 -> Product2/1
  CO+1/2O2->CO2/1 -> Product1/2
  Selector1/1 -> Product1/1
  C+O2->CO2/1 -> Product/2
  burnt_compsition/1(b_comp) -> b_comp/1, Subtract/1
  cal_af/1(af) -> Saturation/1, burnt_compsition/1(af)
  cyl_gas/1 -> init_gas/1, burnt_compsition/2(mol_su), Subtract/2, cal_af/1(cyl_gas)
  Product/1 -> Add/1
  Product1/1 -> Add/2
  Product2/1 -> Add/3
  H+1/2O2->H2O1/1 -> Product3/2
  Selector3/1 -> Product3/1
  Product3/1 -> Add/4
  H/C/1 -> Product3/3
  Saturation/1 -> af/1
  Selector4/1 -> Product/1

== system benchmark_model/ENGINE/engine_s/cylinders/cyl1/cyl/frame/ratio_burnt1/mod720(u,4*pi) ==
  u : Inport
  Constant7 : Constant  Value=4*pi
  Math Function : Math  Operator=mod  SignedPower=on  SaturateOnIntegerOverflow=on
  y : Outport
  wires:
  Math Function/1 -> y/1
  u/1 -> Math Function/1
  Constant7/1 -> Math Function/2

== system benchmark_model/ENGINE/engine_s/cylinders/cyl1/cyl/frame/ratio_burnt1/murnt_ratio ==
  u : Inport
  SA : Inport  Port=2
  rps : Inport  Port=3
  KL : Inport  Port=4
  AF : Inport  Port=5
  EGR : Inport  Port=6
  VT : Inport  Port=7
  Constant2 : Constant  Value=2
  Constant6 : Constant  Value=6
  Embedded MATLAB Function : MATLAB Function  TreatAsAtomicUnit=on
  Gain1 : Gain  Gain=2
  Gain2 : Gain  Gain=180/pi
  Gain3 : Gain  Gain=pi/180
  Mux : Mux
  Phi050 DoE model : Subsystem
  q : Outport
  Q : Outport  Port=2
  wires:
  Gain3/1 -> Mux/4
  Embedded MATLAB Function/1(q) -> q/1
  SA/1 -> Gain3/1, Phi050 DoE model/3(SA)
  Mux/1 -> Embedded MATLAB Function/2(Web)
  Constant6/1 -> Mux/1
  Constant2/1 -> Mux/2
  Phi050 DoE model/1(Phi50) -> Gain1/1
  rps/1 -> Phi050 DoE model/1(N)
  KL/1 -> Phi050 DoE model/2(KL)
  VT/1 -> Gain2/1
  AF/1 -> Phi050 DoE model/5(AFR)
  Gain1/1 -> Mux/3
  EGR/1 -> Phi050 DoE model/6(EGR)
  u/1 -> Embedded MATLAB Function/1(u)
  Embedded MATLAB Function/2(Q) -> Q/1
  Gain2/1 -> Phi050 DoE model/4(VVT)

== system benchmark_model/ENGINE/engine_s/cylinders/cyl1/cyl/knock_Integral/Subsystem1/Subsystem ==
  Tu : Inport
  Constant1 : Constant  Value=FR_C3
  Divide : Product  Inputs=/*
  Math Function1 : Math  SignedPower=on  SaturateOnIntegerOverflow=on
  Saturation : Saturate  UpperLimit=inf  LowerLimit=1.0e-5
  Out1 : Outport
  wires:
  Constant1/1 -> Divide/2
  Divide/1 -> Math Function1/1
  Math Function1/1 -> Out1/1
  Tu/1 -> Saturation/1
  Saturation/1 -> Divide/1

== system benchmark_model/ENGINE/engine_s/cylinders/cyl1/cyl/knock_Integral/Subsystem1/cal_unburned_temp ==
  Pc : Inport
  Tc : Inport  Port=2
  trg_inc : Inport  Port=3
  Constant : Constant  Value=1-1/Kex
  Divide3 : Product  Inputs=*/
  Divide4 : Product
  Math Function2 : Math  Operator=pow  SignedPower=on  SaturateOnIntegerOverflow=on
  Subsystem : Subsystem
  Tu : Outport
  wires:
  Subsystem/1(Pc_inc) -> Divide3/2
  Divide3/1 -> Math Function2/1
  Math Function2/1 -> Divide4/1
  Subsystem/2(Tc_inc) -> Divide4/2
  Constant/1 -> Math Function2/2
  Divide4/1 -> Tu/1
  Tc/1 -> Subsystem/2(Tc)
  Pc/1 -> Subsystem/1(Pc), Divide3/1
  trg_inc/1 -> Subsystem/Trigger

== system benchmark_model/ENGINE/engine_s/cylinders/cyl2/cyl/Energy_Int/dvol/func_d_cylvol(u,SPEC) ==
  In1 : Inport
  Constant1 : Constant  Value=SPEC
  Embedded MATLAB Function1 : MATLAB Function  TreatAsAtomicUnit=on
  Out1 : Outport
  wires:
  Embedded MATLAB Function1/1(y) -> Out1/1
  In1/1 -> Embedded MATLAB Function1/1(u)
  Constant1/1 -> Embedded MATLAB Function1/2(SPEC)

== system benchmark_model/ENGINE/engine_s/cylinders/cyl2/cyl/frame/Init_cyl_gas/capture_cyl_state ==
  cyl_gas : Inport
  Trigger : TriggerPort  VariantControl=(inherit)
  Add : Sum  Inputs=++++
  C+O2->CO2 : Constant  Value=4.19*97200.0
  CO+1/2O2->CO2 : Constant  Value=4.19*29620.0
  H+1/2O2->H2O : Constant  Value=4.19*57750.0
  H+1/2O2->H2O1 : Constant  Value=4.19*57750.0
  H/C : Constant  Value=y/2
  Product : Product  RndMeth=Zero
  Product1 : Product  RndMeth=Zero
  Product2 : Product  RndMeth=Zero
  Product3 : Product  Inputs=3  RndMeth=Zero
  Saturation : Saturate  UpperLimit=22  LowerLimit=6
  Selector1 : Selector  InputPortWidth=7  IndexOptions=Index vector (dialog)  Indices=[3]  OutputSizes=[(-2)]
  Selector2 : Selector  InputPortWidth=7  IndexOptions=Index vector (dialog)  Indices=[5]  OutputSizes=[(-2)]
  Selector3 : Selector  InputPortWidth=7  IndexOptions=Index vector (dialog)  Indices=[1]  OutputSizes=[(-2)]
  Selector4 : Selector  InputPortWidth=7  IndexOptions=Index vector (dialog)  Indices=[1]  OutputSizes=[(-2)]
  Subtract : Sum  Inputs=-+
  burnt_compsition : Subsystem
  cal_af : Subsystem
  Qmax : Outport
  b_comp : Outport  Port=2  InitialOutput=[0;0;0;0;0;0;0]
  init_gas : Outport  Port=3  InitialOutput=[0;0;0;0;0;0;0]
  af : Outport  Port=4  InitialOutput=0
  wires:
  Selector4/1 -> Product/1
  Saturation/1 -> af/1
  H/C/1 -> Product3/3
  Product3/1 -> Add/4
  Selector3/1 -> Product3/1
  H+1/2O2->H2O1/1 -> Product3/2
  Product2/1 -> Add/3
  Product1/1 -> Add/2
  Product/1 -> Add/1
  cyl_gas/1 -> cal_af/1(cyl_gas), Subtract/2, burnt_compsition/2(mol_su), init_gas/1
  cal_af/1(af) -> burnt_compsition/1(af), Saturation/1
  burnt_compsition/1(b_comp) -> Subtract/1, b_comp/1
  C+O2->CO2/1 -> Product/2
  Selector1/1 -> Product1/1
  CO+1/2O2->CO2/1 -> Product1/2
  Selector2/1 -> Product2/1
  H+1/2O2->H2O/1 -> Product2/2
  Add/1 -> Qmax/1
  Subtract/1 -> Selector4/1, Selector1/1, Selector2/1, Selector3/1

== system benchmark_model/ENGINE/engine_s/cylinders/cyl2/cyl/frame/ratio_burnt1/mod720(u,4*pi) ==
  u : Inport
  Constant7 : Constant  Value=4*pi
  Math Function : Math  Operator=mod  SignedPower=on  SaturateOnIntegerOverflow=on
  y : Outport
  wires:
  Constant7/1 -> Math Function/2
  u/1 -> Math Function/1
  Math Function/1 -> y/1

== system benchmark_model/ENGINE/engine_s/cylinders/cyl2/cyl/frame/ratio_burnt1/murnt_ratio ==
  u : Inport
  SA : Inport  Port=2
  rps : Inport  Port=3
  KL : Inport  Port=4
  AF : Inport  Port=5
  EGR : Inport  Port=6
  VT : Inport  Port=7
  Constant2 : Constant  Value=2
  Constant6 : Constant  Value=6
  Embedded MATLAB Function : MATLAB Function  TreatAsAtomicUnit=on
  Gain1 : Gain  Gain=2
  Gain2 : Gain  Gain=180/pi
  Gain3 : Gain  Gain=pi/180
  Mux : Mux
  Phi050 DoE model : Subsystem
  q : Outport
  Q : Outport  Port=2
  wires:
  Gain2/1 -> Phi050 DoE model/4(VVT)
  Embedded MATLAB Function/2(Q) -> Q/1
  u/1 -> Embedded MATLAB Function/1(u)
  EGR/1 -> Phi050 DoE model/6(EGR)
  Gain1/1 -> Mux/3
  AF/1 -> Phi050 DoE model/5(AFR)
  VT/1 -> Gain2/1
  KL/1 -> Phi050 DoE model/2(KL)
  rps/1 -> Phi050 DoE model/1(N)
  Phi050 DoE model/1(Phi50) -> Gain1/1
  Constant2/1 -> Mux/2
  Constant6/1 -> Mux/1
  Mux/1 -> Embedded MATLAB Function/2(Web)
  SA/1 -> Phi050 DoE model/3(SA), Gain3/1
  Embedded MATLAB Function/1(q) -> q/1
  Gain3/1 -> Mux/4

== system benchmark_model/ENGINE/engine_s/cylinders/cyl2/cyl/knock_Integral/Subsystem1/Subsystem ==
  Tu : Inport
  Constant1 : Constant  Value=FR_C3
  Divide : Product  Inputs=/*
  Math Function1 : Math  SignedPower=on  SaturateOnIntegerOverflow=on
  Saturation : Saturate  UpperLimit=inf  LowerLimit=1.0e-5
  Out1 : Outport
  wires:
  Saturation/1 -> Divide/1
  Tu/1 -> Saturation/1
  Math Function1/1 -> Out1/1
  Divide/1 -> Math Function1/1
  Constant1/1 -> Divide/2

== system benchmark_model/ENGINE/engine_s/cylinders/cyl2/cyl/knock_Integral/Subsystem1/cal_unburned_temp ==
  Pc : Inport
  Tc : Inport  Port=2
  trg_inc : Inport  Port=3
  Constant : Constant  Value=1-1/Kex
  Divide3 : Product  Inputs=*/
  Divide4 : Product
  Math Function2 : Math  Operator=pow  SignedPower=on  SaturateOnIntegerOverflow=on
  Subsystem : Subsystem
  Tu : Outport
  wires:
  trg_inc/1 -> Subsystem/Trigger
  Pc/1 -> Divide3/1, Subsystem/1(Pc)
  Tc/1 -> Subsystem/2(Tc)
  Divide4/1 -> Tu/1
  Constant/1 -> Math Function2/2
  Subsystem/2(Tc_inc) -> Divide4/2
  Math Function2/1 -> Divide4/1
  Divide3/1 -> Math Function2/1
  Subsystem/1(Pc_inc) -> Divide3/2

== system benchmark_model/ENGINE/engine_s/cylinders/cyl3/cyl/Energy_Int/dvol/func_d_cylvol(u,SPEC) ==
  In1 : Inport
  Constant1 : Constant  Value=SPEC
  Embedded MATLAB Function1 : MATLAB Function  TreatAsAtomicUnit=on
  Out1 : Outport
  wires:
  Constant1/1 -> Embedded MATLAB Function1/2(SPEC)
  In1/1 -> Embedded MATLAB Function1/1(u)
  Embedded MATLAB Function1/1(y) -> Out1/1
